simulink model "KinematicWheelWith6DOF"  (R2017b)
settings: Solver=VariableStepAuto  StartTime=0.0  StopTime=5  RelTol=1e-3  EnableMultiTasking=on
undefined symbols (not defined in the file): radiusRW, X, Y, Z
libraries: nesl_utility x16, sm_lib x7, Contact_Forces_Lib x7, Parts_Lib x1, vrlib x1, simulink x1
settings Model: Creator=rizwan  LastModifiedBy=r_ahmed_afzal
settings DataIOCC: LimitDataPoints=on
settings OptimizationCC: LifeSpan=inf
settings DebuggingCC: AllowSymbolicDim=off  SFUnexpectedBacktrackingDiag=warning  SFNoUnconditionalDefaultTransitionDiag=warning  SFExecutionAtInitializationDiag=none
settings CodeAppCC: StateflowObjectComments=on
settings GRTTargetCC: TargetLangStandard=C89/C90 (ANSI)  GeneratePreprocessorConditionals=Disable all
settings ConfigComp: CovMetricSettings=dw  CovHtmlReporting=on  CovSaveCumulativeToWorkspaceVar=on  CovSaveSingleToWorkspaceVar=on  CovExternalEMLEnable=off  CovSFcnEnable=off
settings SimscapeCC: SimscapeNominalValues="[{\"value\":\"10\",\"unit\":\"V\"},{\"value\":\"1\",\"unit\":\"A\"},{\"value\":\"10\",\"unit\":\"N*m\"},{\"value\":\"10\",\"unit\":\"bar\"},{\"value\":\"100\",\"unit\":\"kJ/kg\"},{\"value\":\"1\",\"unit\":\"kW\"},{\"value\":\"300\",\"unit\":\"K\"},{\"value\":\"100\",\"unit\":\"cm^3/s\"},{\"value\":\"1\",\"unit\":\"kN\"},{\"value\":\"1\",\"unit\":\"g/cm^3\"},{\"value\":\"1\",\"unit\":\"l\"},{\"value\":\"1\",\"unit\":\"cm^2\"},{\"value\":\"60\",\"unit\":\"Hz\"}]"  SimscapeLogType=all  SimscapeLogDataHistory=10000
settings ConfigurationSet: Description=SimMechanics 2G

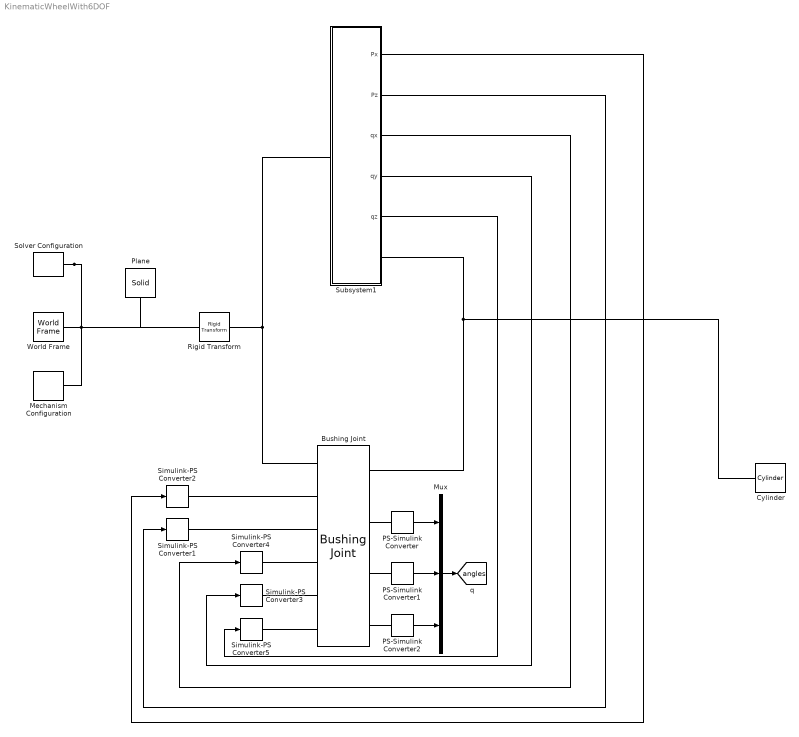
== system KinematicWheelWith6DOF ==
  Bushing Joint : sm_lib/Joints/Bushing Joint  SenseConstraintForce=off  SenseConstraintForceX=off  SenseConstraintForceY=off  SenseConstraintForceZ=off  SenseConstraintTorque=off  SenseConstraintTorqueX=off  SenseConstraintTorqueY=off  SenseConstraintTorqueZ=off  SenseTotalForce=off  SenseTotalForceX=off  SenseTotalForceY=off  SenseTotalForceZ=off  SenseTotalTorque=off  SenseTotalTorqueX=off  SenseTotalTorqueY=off  SenseTotalTorqueZ=off  CompositeWrenchDir=FollowerOnBase  CompositeWrenchFrame=BaseFrame  PxEquilibriumPosition=0  PxEquilibriumPositionUnits=m  PxSpringStiffness=0  PxSpringStiffnessUnits=N/m  PxDampingCoefficient=0  PxDampingCoefficientUnits=N/(m/s)  PxTorqueActuationMode=ComputedTorque  PxMotionActuationMode=InputMotion  PxSensePosition=off  PxSenseVelocity=off  PxSenseAcceleration=off  PxSenseTorqueForce=off  PxPositionTargetSpecify=off  PxPositionTargetPriority=High  PxPositionTargetValue=0  PxPositionTargetValueUnits=m  PxVelocityTargetSpecify=off  PxVelocityTargetPriority=High  PxVelocityTargetValue=0  PxVelocityTargetValueUnits=m/s  PyEquilibriumPosition=0  PyEquilibriumPositionUnits=m  PySpringStiffness=0  PySpringStiffnessUnits=N/m  PyDampingCoefficient=0  PyDampingCoefficientUnits=N/(m/s)  PyTorqueActuationMode=NoTorque  PyMotionActuationMode=ComputedMotion  PySensePosition=off  PySenseVelocity=off  PySenseAcceleration=off  PySenseTorqueForce=off  PyPositionTargetSpecify=on  PyPositionTargetPriority=High  PyPositionTargetValue=-radiusRW  PyPositionTargetValueUnits=m  PyVelocityTargetSpecify=off  PyVelocityTargetPriority=High  PyVelocityTargetValue=0  PyVelocityTargetValueUnits=m/s  PzEquilibriumPosition=0  PzEquilibriumPositionUnits=m  PzSpringStiffness=0  PzSpringStiffnessUnits=N/m  PzDampingCoefficient=0  PzDampingCoefficientUnits=N/(m/s)  PzTorqueActuationMode=ComputedTorque  PzMotionActuationMode=InputMotion  PzSensePosition=off  PzSenseVelocity=off  PzSenseAcceleration=off  PzSenseTorqueForce=off  PzPositionTargetSpecify=off  PzPositionTargetPriority=High  PzPositionTargetValue=0  PzPositionTargetValueUnits=m  PzVelocityTargetSpecify=off  PzVelocityTargetPriority=High  PzVelocityTargetValue=0  PzVelocityTargetValueUnits=m/s  RxEquilibriumPosition=0  RxEquilibriumPositionUnits=deg  RxSpringStiffness=0  RxSpringStiffnessUnits=N*m/deg  RxDampingCoefficient=0  RxDampingCoefficientUnits=N*m/(deg/s)  RxTorqueActuationMode=ComputedTorque  RxMotionActuationMode=InputMotion  RxSensePosition=on  RxSenseVelocity=off  RxSenseAcceleration=off  RxSenseTorqueForce=off  RxPositionTargetSpecify=off  RxPositionTargetPriority=High  RxPositionTargetValue=0  RxPositionTargetValueUnits=deg  RxVelocityTargetSpecify=off  RxVelocityTargetPriority=High  RxVelocityTargetValue=0  RxVelocityTargetValueUnits=deg/s  RyEquilibriumPosition=0  RyEquilibriumPositionUnits=deg  RySpringStiffness=0  RySpringStiffnessUnits=N*m/deg  RyDampingCoefficient=0  RyDampingCoefficientUnits=N*m/(deg/s)  RyTorqueActuationMode=ComputedTorque  RyMotionActuationMode=InputMotion  RySensePosition=on  RySenseVelocity=off  RySenseAcceleration=off  RySenseTorqueForce=off  RyPositionTargetSpecify=off  RyPositionTargetPriority=High  RyPositionTargetValue=0  RyPositionTargetValueUnits=deg  RyVelocityTargetSpecify=off  RyVelocityTargetPriority=High  RyVelocityTargetValue=0  RyVelocityTargetValueUnits=deg/s  RzEquilibriumPosition=0  RzEquilibriumPositionUnits=deg  RzSpringStiffness=0  RzSpringStiffnessUnits=N*m/deg  RzDampingCoefficient=0  RzDampingCoefficientUnits=N*m/(deg/s)  RzTorqueActuationMode=ComputedTorque  RzMotionActuationMode=InputMotion  RzSensePosition=on  RzSenseVelocity=off  RzSenseAcceleration=off  RzSenseTorqueForce=off  RzPositionTargetSpecify=off  RzPositionTargetPriority=High  RzPositionTargetValue=0  RzPositionTargetValueUnits=deg  RzVelocityTargetSpecify=off  RzVelocityTargetPriority=High  RzVelocityTargetValue=0  RzVelocityTargetValueUnits=deg/s
      settings: SourceProductName=Simscape Multibody
  Cylinder : Parts_Lib/Cylinder  Tag=CustomStyle  cyl_radius=radiusRW  cyl_length=lengthRW  cyl_density=rhoRW  cyl_color=blue  cyl_opacity=1  cyl_color_custom="[0.7920    0.9900    0.9900]"  mark_radius=[0.75 0.5]  mark_len_factor=1.01  mark_angle=60  mark_color=purple  mark_opacity=1
  Mechanism Configuration : sm_lib/Utilities/Mechanism Configuration  UniformGravity=Constant  GravityVector=[0 0 -0]  GravityUnits=m/s^2  LinearizationDelta=0.001
  Mux : Mux  Inputs=3
  PS-Simulink Converter : nesl_utility/PS-Simulink Converter  PhysicalDomain=network_engine_domain  SubClassName=ps_output  LeftPortType=input  RightPortType=output  PseudoPeriodic=off  Frequencies=[]  Unit=1  AffineConversion=off
  PS-Simulink Converter1 : nesl_utility/PS-Simulink Converter  PhysicalDomain=network_engine_domain  SubClassName=ps_output  LeftPortType=input  RightPortType=output  PseudoPeriodic=off  Frequencies=[]  Unit=1  AffineConversion=off
  PS-Simulink Converter2 : nesl_utility/PS-Simulink Converter  PhysicalDomain=network_engine_domain  SubClassName=ps_output  LeftPortType=input  RightPortType=output  PseudoPeriodic=off  Frequencies=[]  Unit=1  AffineConversion=off
  Plane : sm_lib/Body Elements/Solid  InertiaType=CalculateFromGeometry  Mass=1  MassUnits=kg  CenterOfMass=[0 0 0]  CenterOfMassUnits=m  MomentsOfInertia=[1 1 1]  MomentsOfInertiaUnits=kg*m^2  ProductsOfInertia=[1 1 1]  ProductsOfInertiaUnits=kg*m^2  DensityBased=on  Density=1000  DensityUnits=kg/m^3  DoExposeReferenceFrame=on  SerializedFrames=<Frames/>  GraphicType=FromGeometry  MarkerShape=Sphere  MarkerSize=10  GraphicVisPropType=SimpleVisualProperties  GraphicDiffuseColor=[0.5 0.5 0.5]  GraphicSpecularColor=[0.5 0.5 0.5 1.0]  GraphicAmbientColor=[0.15 0.15 0.15 1.0]  GraphicEmissiveColor=[0.0 0.0 0.0 1.0]  GraphicShininess=75  GraphicOpacity=0.5  GeometryShape=Brick  RectangleSize=[1 1]  RectangleSizeUnits=m  BrickDimensions=[10 4 0.01]  BrickDimensionUnits=m  CylinderRadius=1  CylinderRadiusUnits=m  CylinderLength=1  CylinderLengthUnits=m  SphereRadius=1  SphereRadiusUnits=m  EllipsoidRadii=[1 1 1]  EllipsoidRadiiUnits=m  ExtrusionCrossSection=[1 1; -1 1; -1 -1; 1 -1]  ExtrusionCrossSectionUnits=m  ExtrusionLength=1  ExtrusionLengthUnits=m  PolygonNumSides=3  PolygonOuterRadius=1  PolygonOuterRadiusUnits=m  ExtGeomFileType=STEP  ExtGeomFileUnits=m  RevolutionCrossSection=[1 1; 1 -1; 2 -1; 2 1]  RevolutionCrossSectionUnits=m  RevolutionExtent=Full  RevolutionAngle=180  RevolutionAngleUnits=deg
  Rigid Transform : sm_lib/Frames and Transforms/Rigid Transform  TranslationMethod=None  TranslationStandardOffset=0  TranslationLengthUnit=m  TranslationStandardAxis=+Z  TranslationCartesianOffset=[0 0 0]  TranslationROffset=0  TranslationROffsetUnits=m  TranslationZOffset=0  TranslationZOffsetUnits=m  TranslationThetaOffset=0  TranslationThetaOffsetUnits=deg  RotationMethod=AlignedAxes  RotationAngleUnits=deg  RotationStandardAxis=+Z  RotationAngle=0.0  RotationArbitraryAxis=[0 0 1]  FollAlignAxisA=+Z  BaseAlignAxisA=+Y  FollAlignAxisB=+X  BaseAlignAxisB=+X  RotationSequenceAxes=FollowerAxes  RotationSequence=XYX  RotationSequenceAngles=[0 0 0]  RotationSequenceAnglesUnits=deg  RotationMatrix=[1 0 0; 0 1 0; 0 0 1]
  Simulink-PS Converter{1..5} (5 alike) : nesl_utility/Simulink-PS Converter  PhysicalDomain=network_engine_domain  SubClassName=ps_input  LeftPortType=input  RightPortType=output  PseudoPeriodic=off  Frequencies=[]  NoiseDistribution=none  NoiseParameters=[]  Unit=1  AffineConversion=off  FilteringAndDerivatives=filter  SimscapeFilterOrder=2  InputFilterTimeConstant=0.001  UdotUserProvided=0
  Solver Configuration : nesl_utility/Solver Configuration  PhysicalDomain=network_engine_domain  SubClassName=solver  LeftPortType=input  RightPortType=generic  Accelerate=off  Tones=[]  Harmonics=[]  SimulateNoise=off  Profile=off  UseLocalSampling=off  EnableSwitchedLinearOptims=on  FrequencyDomain=off  UseCCode=off  RelTol=0.001  AbsTol=1e-06  MinStep=1e-09  ToWorkspace=off  RevertToSquareIcSolve=off  NumHomotopyIterations=100  PhasorMode=off  PhasorModeNumHarmonics=1  DoDC=off  ResidualTolerance=1e-09  UseLocalSolver=off  LocalSolverChoice=NE_BACKWARD_EULER_ADVANCER  LocalSolverSampleTime=0.001  DoFixedCost=off  MaxNonlinIter=3  MaxModeIter=2  LinearAlgebra=Sparse  DelaysMemoryBudget=1024  AutomaticFiltering=on  FilteringTimeConstant=0.001
  Subsystem1 : Subsystem
  World Frame : sm_lib/Frames and Transforms/World Frame
  tag scope: angles=global
  wires:
  Subsystem1/1(Px) -> Simulink-PS Converter2/1
  Subsystem1/2(Pz) -> Simulink-PS Converter1/1
  Subsystem1/4(qy) -> Simulink-PS Converter3/1
  Subsystem1/3(qx) -> Simulink-PS Converter4/1
  Subsystem1/5(qz) -> Simulink-PS Converter5/1
  PS-Simulink Converter1/1 -> Mux/2
  PS-Simulink Converter/1 -> Mux/1
  PS-Simulink Converter2/1 -> Mux/3
  Mux/1 -> [angles]
  connections:
  Solver Configuration/RConn1 -- Rigid Transform/LConn1 -- Plane/RConn1 -- Mechanism Configuration/RConn1 -- World Frame/RConn1
  Subsystem1/RConn1 -- Bushing Joint/RConn1 -- Cylinder/LConn1
  Subsystem1/LConn1 -- Bushing Joint/LConn1 -- Rigid Transform/RConn1
  Bushing Joint/LConn2 -- Simulink-PS Converter2/RConn1
  Simulink-PS Converter1/RConn1 -- Bushing Joint/LConn3
  Simulink-PS Converter3/RConn1 -- Bushing Joint/LConn5
  Simulink-PS Converter4/RConn1 -- Bushing Joint/LConn4
  Simulink-PS Converter5/RConn1 -- Bushing Joint/LConn6
  PS-Simulink Converter/LConn1 -- Bushing Joint/RConn2
  PS-Simulink Converter1/LConn1 -- Bushing Joint/RConn3
  PS-Simulink Converter2/LConn1 -- Bushing Joint/RConn4

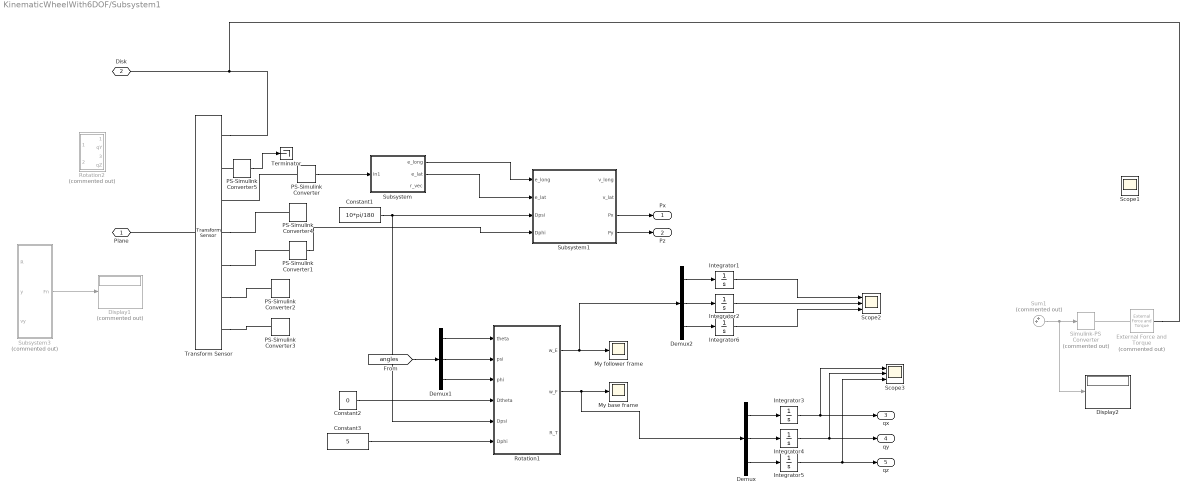
== system KinematicWheelWith6DOF/Subsystem1 ==
  Constant1 : Constant  Value=10*pi/180
  Constant2 : Constant  Value=0
  Constant3 : Constant  Value=5
  Demux : Demux  Outputs=3
  Demux1 : Demux  Outputs=3
  Demux2 : Demux  Outputs=3
  Display1 : Display  Commented=on
  Display2 : Display
  External Force and Torque : sm_lib/Forces and Torques/External Force and Torque  Commented=on  ForceResolutionFrame=AttachedFrame  EnableForceX=off  EnableForceY=off  EnableForceZ=off  EnableForce=on  TorqueResolutionFrame=AttachedFrame  EnableTorqueX=off  EnableTorqueY=off  EnableTorqueZ=off  EnableTorque=off
  Integrator{1..6} (6 alike) : Integrator
  My base frame : Scope
  My follower frame : Scope
  PS-Simulink Converter{,1..5} (6 alike) : nesl_utility/PS-Simulink Converter  PhysicalDomain=network_engine_domain  SubClassName=ps_output  LeftPortType=input  RightPortType=output  PseudoPeriodic=off  Frequencies=[]  Unit=1  AffineConversion=off
  Rotation1 : MATLAB Function  TreatAsAtomicUnit=on
  Rotation2 : Subsystem  Commented=on
  Scope1 : Scope
  Scope2 : Scope  NumInputPorts=3
  Scope3 : Scope  NumInputPorts=3
  Simulink-PS Converter : nesl_utility/Simulink-PS Converter  Commented=on  PhysicalDomain=network_engine_domain  SubClassName=ps_input  LeftPortType=input  RightPortType=output  PseudoPeriodic=off  Frequencies=[]  NoiseDistribution=none  NoiseParameters=[]  Unit=1  AffineConversion=off  FilteringAndDerivatives=filter  SimscapeFilterOrder=2  InputFilterTimeConstant=0.001  UdotUserProvided=0
  Subsystem : Subsystem
  Subsystem1 : Subsystem
  Subsystem3 : Subsystem  Commented=on
  Sum1 : Sum  Commented=on  Inputs=++|
  Terminator : Terminator
  Transform Sensor : sm_lib/Frames and Transforms/Transform Sensor  MeasurementFrame=Base  SenseAngle=on  SenseAxis=off  SenseAngle1=off  SenseAngle2=off  SenseAngle3=off  SenseQ=off  SenseR=on  SenseOmegaX=off  SenseOmegaY=on  SenseOmegaZ=on  SenseOmega1=off  SenseOmega2=off  SenseOmega3=off  SenseQDot=off  SenseRDot=off  SenseAlphaX=off  SenseAlphaY=off  SenseAlphaZ=off  SenseAlpha1=off  SenseAlpha2=off  SenseAlpha3=off  SenseQDDot=off  SenseRDDot=off  SenseX=off  SenseY=on  SenseZ=off  SenseRad=off  SenseAzim=off  SenseDist=off  SenseInc=off  SenseXDot=off  SenseYDot=on  SenseZDot=off  SenseRadDot=off  SenseAzimDot=off  SenseDistDot=off  SenseIncDot=off  SenseXDDot=off  SenseYDDot=off  SenseZDDot=off  SenseRadDDot=off  SenseAzimDDot=off  SenseDistDDot=off  SenseIncDDot=off
  Plane : PMIOPort  Port=1  Side=Left
  Disk : PMIOPort  Port=2  Side=Right
  Px : Outport
  Pz : Outport  Port=2
  qx : Outport  Port=3
  qy : Outport  Port=4
  qz : Outport  Port=5
  wires:
  PS-Simulink Converter/1 -> Subsystem/1(In1)
  Subsystem/1(e_long) -> Subsystem1/1(e_long)
  Subsystem/2(e_lat) -> Subsystem1/2(e_lat)
  Constant1/1 -> Rotation1/5(Dpsi), Subsystem1/3(Dpsi)
  Subsystem1/3(Px) -> Px/1
  Subsystem1/4(Py) -> Pz/1
  Subsystem3/1(Fn) -> Display1/1
  Sum1/1 -> Display2/1, Simulink-PS Converter/1
  PS-Simulink Converter1/1 -> Subsystem1/4(Dphi)
  Constant2/1 -> Rotation1/4(Dtheta)
  Rotation1/2(w_F) -> Demux/1, My base frame/1
  Demux/2 -> Integrator4/1
  Demux/1 -> Integrator3/1
  Demux/3 -> Integrator5/1
  Constant3/1 -> Rotation1/6(Dphi)
  Integrator3/1 -> Scope3/1, qx/1
  Integrator4/1 -> Scope3/2, qy/1
  Integrator5/1 -> Scope3/3, qz/1
  [angles] -> Demux1/1
  Demux1/1 -> Rotation1/1(theta)
  Demux1/2 -> Rotation1/2(psi)
  Demux1/3 -> Rotation1/3(phi)
  PS-Simulink Converter5/1 -> Terminator/1
  Demux2/3 -> Integrator6/1
  Integrator2/1 -> Scope2/2
  Integrator6/1 -> Scope2/3
  Demux2/1 -> Integrator1/1
  Integrator1/1 -> Scope2/1
  Demux2/2 -> Integrator2/1
  Rotation1/1(w_E) -> Demux2/1, My follower frame/1
  connections:
  Transform Sensor/RConn1 -- External Force and Torque/RConn1 -- Disk/RConn1
  Transform Sensor/LConn1 -- Plane/RConn1
  External Force and Torque/LConn1 -- Simulink-PS Converter/RConn1
  PS-Simulink Converter/LConn1 -- Transform Sensor/RConn3
  Transform Sensor/RConn4 -- PS-Simulink Converter4/LConn1
  Transform Sensor/RConn5 -- PS-Simulink Converter1/LConn1
  Transform Sensor/RConn6 -- PS-Simulink Converter2/LConn1
  Transform Sensor/RConn7 -- PS-Simulink Converter3/LConn1
  PS-Simulink Converter5/LConn1 -- Transform Sensor/RConn2

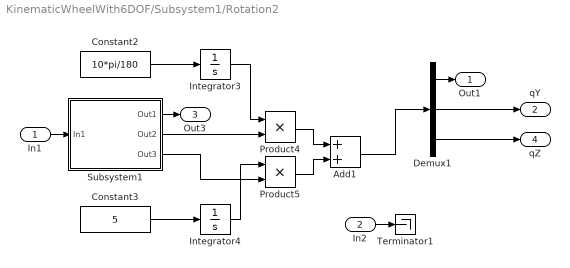
== system KinematicWheelWith6DOF/Subsystem1/Rotation2 ==
  In1 : Inport
  In2 : Inport  Port=2
  Add1 : Sum
  Constant2 : Constant  Value=10*pi/180
  Constant3 : Constant  Value=5
  Demux1 : Demux  Outputs=3
  Integrator3 : Integrator
  Integrator4 : Integrator
  Product4 : Product
  Product5 : Product
  Subsystem1 : Subsystem
  Terminator1 : Terminator
  Out1 : Outport
  qY : Outport  Port=2
  Out3 : Outport  Port=3
  qZ : Outport  Port=4
  wires:
  Demux1/1 -> Out1/1
  Subsystem1/1(Out1) -> Out3/1
  In1/1 -> Subsystem1/1(In1)
  In2/1 -> Terminator1/1
  Constant2/1 -> Integrator3/1
  Demux1/2 -> qY/1
  Constant3/1 -> Integrator4/1
  Integrator3/1 -> Product4/1
  Integrator4/1 -> Product5/1
  Product4/1 -> Add1/1
  Subsystem1/3(Out3) -> Product5/2
  Add1/1 -> Demux1/1
  Demux1/3 -> qZ/1
  Product5/1 -> Add1/2
  Subsystem1/2(Out2) -> Product4/2

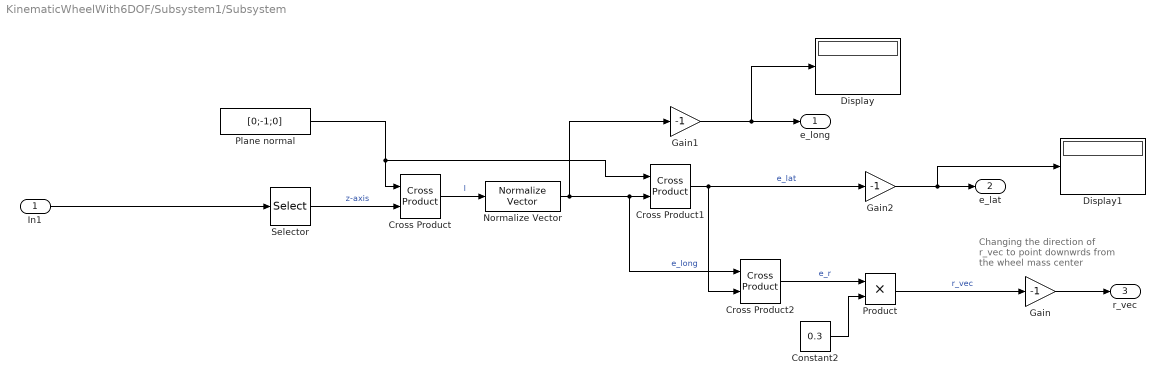
== system KinematicWheelWith6DOF/Subsystem1/Subsystem ==
  note: Changing the direction
      | of r_vec to point downwrds
      | from the wheel mass center
  In1 : Inport
  Constant2 : Constant  Value=0.3
  Cross Product : Contact_Forces_Lib/Math/Cross Product
  Cross Product1 : Contact_Forces_Lib/Math/Cross Product
  Cross Product2 : Contact_Forces_Lib/Math/Cross Product
  Display : Display
  Display1 : Display
  Gain : Gain  Gain=-1
  Gain1 : Gain  Gain=-1
  Gain2 : Gain  Gain=-1
  Normalize Vector : vrlib/Utilities/Normalize Vector  maxzero=0
      settings: SourceProductName=Simulink 3D Animation  SourceProductBaseCode=VR
  Plane normal : Constant  Value=[0;-1;0]
  Product : Product
  Selector : Selector  NumberOfDimensions=2  InputPortWidth=3  IndexOptions=Index vector (dialog),Index vector (dialog)  Indices=[1:3],3  OutputSizes=1,1
  e_long : Outport
  e_lat : Outport  Port=2
  r_vec : Outport  Port=3
  wires:
  Constant2/1 -> Product/2
  Product/1 -> Gain/1  "r_vec"
  Cross Product2/1 -> Product/1  "e_r"
  Normalize Vector/1 -> Gain1/1, Cross Product2/1, Cross Product1/2  "e_long"
  Cross Product1/1 -> Gain2/1, Cross Product2/2  "e_lat"
  Selector/1 -> Cross Product/2  "z-axis"
  Cross Product/1 -> Normalize Vector/1  "l"
  In1/1 -> Selector/1
  Plane normal/1 -> Cross Product/1, Cross Product1/1
  Gain/1 -> r_vec/1
  Gain1/1 -> Display/1, e_long/1
  Gain2/1 -> Display1/1, e_lat/1

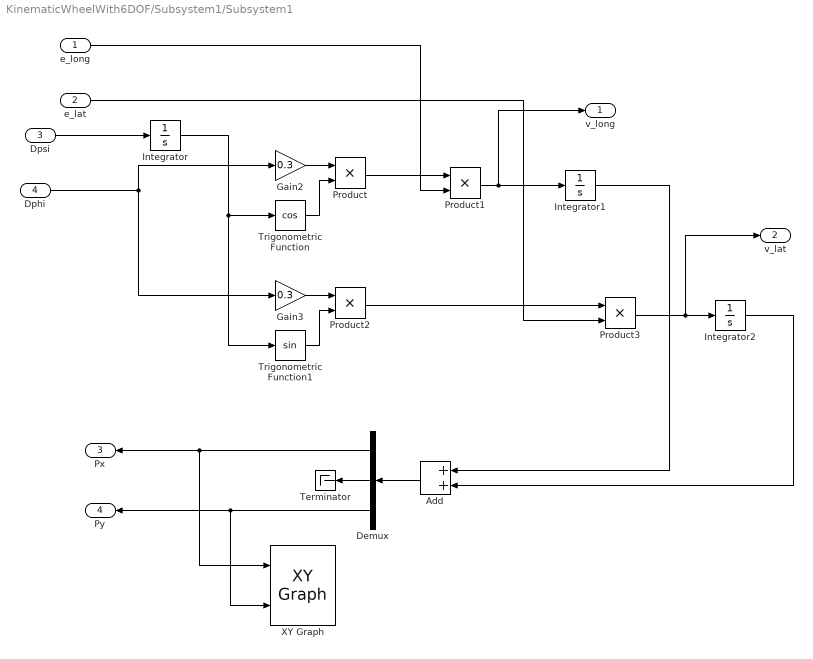
== system KinematicWheelWith6DOF/Subsystem1/Subsystem1 ==
  e_long : Inport
  e_lat : Inport  Port=2
  Dpsi : Inport  Port=3
  Dphi : Inport  Port=4
  Add : Sum  Inputs=2
  Demux : Demux  Outputs=3
  Gain2 : Gain  Gain=0.3
  Gain3 : Gain  Gain=0.3
  Integrator : Integrator
  Integrator1 : Integrator
  Integrator2 : Integrator
  Product{,1..3} (4 alike) : Product
  Terminator : Terminator
  Trigonometric Function : Trigonometry  Operator=cos
  Trigonometric Function1 : Trigonometry
  XY Graph : simulink/Sinks/XY Graph  xmin=0  xmax=7  ymin=0  ymax=7  st=-1
  v_long : Outport
  v_lat : Outport  Port=2
  Px : Outport  Port=3
  Py : Outport  Port=4
  wires:
  Dphi/1 -> Gain2/1, Gain3/1
  Dpsi/1 -> Integrator/1
  Integrator1/1 -> Add/1
  Demux/1 -> Px/1, XY Graph/1
  Demux/2 -> Terminator/1
  e_long/1 -> Product1/2
  Add/1 -> Demux/1
  Integrator2/1 -> Add/2
  Demux/3 -> Py/1, XY Graph/2
  e_lat/1 -> Product3/2
  Product/1 -> Product1/1
  Gain2/1 -> Product/1
  Trigonometric Function/1 -> Product/2
  Trigonometric Function1/1 -> Product2/2
  Gain3/1 -> Product2/1
  Integrator/1 -> Trigonometric Function1/1, Trigonometric Function/1
  Product1/1 -> v_long/1, Integrator1/1
  Product2/1 -> Product3/1
  Product3/1 -> v_lat/1, Integrator2/1

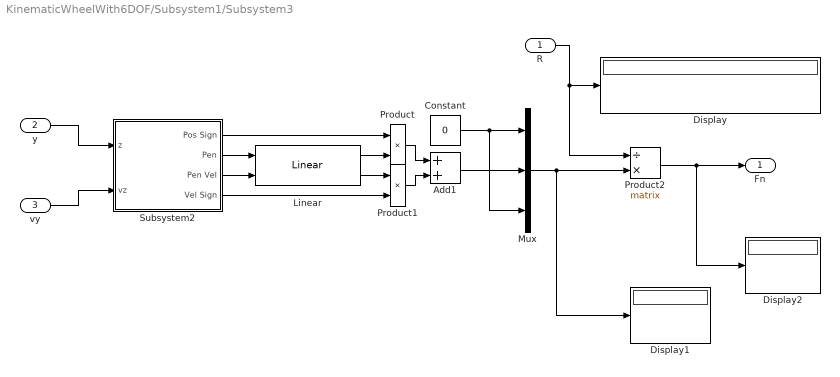
== system KinematicWheelWith6DOF/Subsystem1/Subsystem3 ==
  R : Inport
  y : Inport  Port=2
  vy : Inport  Port=3
  Add1 : Sum
  Constant : Constant  Value=0
  Display : Display
  Display1 : Display
  Display2 : Display
  Linear : Contact_Forces_Lib/Force Law/Linear  VariantControl=Linear  k_pen=1e5  b_penvel=2e3
  Mux : Mux  Inputs=3
  Product : Product
  Product1 : Product
  Product2 : Product  Inputs=/*  Multiplication=Matrix(*)
  Subsystem2 : Subsystem
  Fn : Outport
  wires:
  Product/1 -> Add1/1
  Subsystem2/4(Vel Sign) -> Product1/2
  vy/1 -> Subsystem2/2(vz)
  Subsystem2/1(Pos Sign) -> Product/1
  Product1/1 -> Add1/2
  y/1 -> Subsystem2/1(z)
  Linear/1 -> Product/2
  Linear/2 -> Product1/1
  Subsystem2/2(Pen) -> Linear/1
  Subsystem2/3(Pen Vel) -> Linear/2
  Add1/1 -> Mux/2
  Constant/1 -> Mux/3, Mux/1
  R/1 -> Display/1, Product2/1
  Mux/1 -> Display1/1, Product2/2
  Product2/1 -> Display2/1, Fn/1

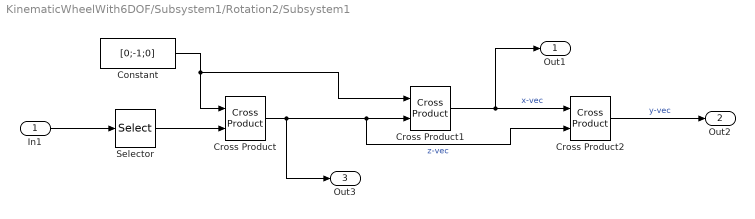
== system KinematicWheelWith6DOF/Subsystem1/Rotation2/Subsystem1 ==
  In1 : Inport
  Constant : Constant  Value=[0;-1;0]
  Cross Product : Contact_Forces_Lib/Math/Cross Product
  Cross Product1 : Contact_Forces_Lib/Math/Cross Product
  Cross Product2 : Contact_Forces_Lib/Math/Cross Product
  Selector : Selector  NumberOfDimensions=2  InputPortWidth=3  IndexOptions=Index vector (dialog),Index vector (dialog)  Indices=[1:3],2  OutputSizes=1,1
  Out1 : Outport
  Out2 : Outport  Port=2
  Out3 : Outport  Port=3
  wires:
  In1/1 -> Selector/1
  Constant/1 -> Cross Product1/1, Cross Product/1
  Selector/1 -> Cross Product/2
  Cross Product/1 -> Out3/1, Cross Product2/2, Cross Product1/2  "z-vec"
  Cross Product1/1 -> Out1/1, Cross Product2/1  "x-vec"
  Cross Product2/1 -> Out2/1  "y-vec"

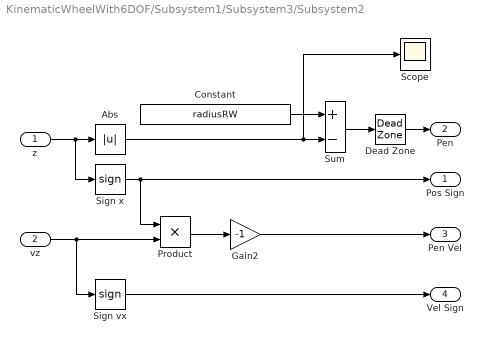
== system KinematicWheelWith6DOF/Subsystem1/Subsystem3/Subsystem2 ==
  z : Inport
  vz : Inport  Port=2
  Abs : Abs  ZeroCross=off
  Constant : Constant  Value=radiusRW
  Dead Zone : DeadZone  LowerValue=-inf  UpperValue=0  SaturateOnIntegerOverflow=on
  Gain2 : Gain  Gain=-1
  Product : Product
  Scope : Scope
  Sign vx : Signum  ZeroCross=off
  Sign x : Signum  ZeroCross=off
  Sum : Sum  Inputs=+-
  Pos Sign : Outport
  Pen : Outport  Port=2
  Pen Vel : Outport  Port=3
  Vel Sign : Outport  Port=4
  wires:
  Gain2/1 -> Pen Vel/1
  Dead Zone/1 -> Pen/1
  Abs/1 -> Scope/1, Sum/2
  Product/1 -> Gain2/1
  Sign vx/1 -> Vel Sign/1
  Sum/1 -> Dead Zone/1
  Constant/1 -> Sum/1
  z/1 -> Sign x/1, Abs/1
  vz/1 -> Product/2, Sign vx/1
  Sign x/1 -> Pos Sign/1, Product/1

== matlab function KinematicWheelWith6DOF/Subsystem1/Rotation1 ==
  data: theta input; w_E output; psi input; phi input; Dtheta input; Dpsi input; Dphi input; w_F output; R_T output
function [w_E,w_F,R_T] = fcn(theta, psi, phi, Dtheta, Dpsi, Dphi)

R1 = [1 0 0;
       0 cos(theta) -sin(theta);
       0 sin(theta) cos(theta)];
   
R2 = [cos(psi) 0 sin(psi);
        0 1 0;
        -sin(psi) 0 cos(psi)];
 
R3 = [cos(phi) -sin(phi) 0;
        sin(phi) cos(phi) 0;
        0 0 1];
    
L1 = transpose(R1);
L2 = transpose(R2);
L3 = transpose(R3);

w_E = (L3*L2*L1)*[Dtheta;0;0] + ...
                 (L3*L2)*[0; Dpsi; 0] + L3*[0; 0; Dphi];
             
% w_F = [Dphi*sin(psi)+Dtheta;
%         -Dphi*sin(theta)*cos(psi)+Dpsi*cos(theta);
%         Dphi*cos(psi)*cos(theta)+Dpsi*sin(theta)];

w_F = R1*R2*R3*w_E;
    
R_T = R1*R2*R3;
end
